simulink model "ME322_Exercise_3_Traction_Motor_Simulink"  (R2024b)
settings: Solver=VariableStepAuto  StartTime=0.0  StopTime=0.025  RelTol=1e-3
undefined symbols (not defined in the file or in its folder): u_trac, x_trac
settings Model: Creator=caidenbonney  LastModifiedBy=Caide

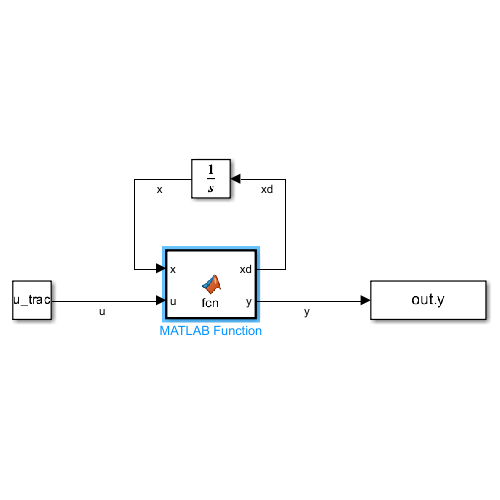
[thumbnail: Simulink's stored preview of the top-level diagram]
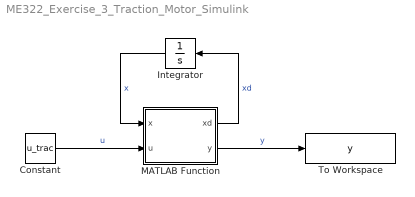
== system ME322_Exercise_3_Traction_Motor_Simulink ==
  Constant : Constant  Value=u_trac  VectorParams1D=off
  Integrator : Integrator  InitialCondition=x_trac
  MATLAB Function : MATLAB Function  TreatAsAtomicUnit=on
  To Workspace : ToWorkspace  VariableName=y  SampleTime=-1
  wires:
  Constant/1 -> MATLAB Function/2(u)  "u"
  MATLAB Function/1(xd) -> Integrator/1  "xd"
  Integrator/1 -> MATLAB Function/1(x)  "x"
  MATLAB Function/2(y) -> To Workspace/1  "y"

== matlab function ME322_Exercise_3_Traction_Motor_Simulink/MATLAB Function ==
  data: x input; xd output size=3; u input; y output size=6; p parameter
function [xd, y]= fcn(x, u, p)

% Separate state variables into individual elements
i_Lm = x(1);     % [A]
omega_Je = x(2); % [rad/sec]
V_me = x(3);    % [m/s]

% Separate input variables into individual elements
v_m = u(1); % [V]

% Required given constants units
p.r_w; % [m]

p.mu_k; % [-]
p.m_e; % [kg]
g = 9.81; % [m/sec^2] (gravity)
p.k; % [-]
p.v_hat; % [m/sec]

p.v_hat; % [m/sec]

p.L_m; % [mH]
L_m = p.L_m *10^-3;  % [mH] -> 10^-3 [H]
p.R_m; % [ohms]
p.K_v; % [V*sec/rad]

p.J_e; % [g/mm^2]
J_e = p.J_e *10^-9;  % [g*mm^2] -> 10^-9 [rad/sec^2)/N*m]^-1
p.K_t; % [N*m/A]
p.b_g; % [N*m/sec]
p.b_m; % [N*m/sec]
p.r_w; % [m]

p.m_e; % [kg]

% Output Equations
V_btr = p.r_w*omega_Je - V_me; % [m/sec]

F_max = p.mu_k*p.m_e*g; % [N]
F_btr = ((2*F_max)/pi)*atan((tan((pi*p.k)/2)/p.v_hat)*V_btr); % [N]

alpha_btr = abs(V_btr) >= p.v_hat; % [-]

% State Equations
id_Lm = (1/(L_m))*(v_m - p.R_m*i_Lm - p.K_v*(p.N_G/p.N_P)*omega_Je); % <-- State eq. f_1
    % the expected units of the derivative of current with respect to
    % time is [A/sec]
        % (1/[H])    *    ([V] - [ohms]*[A] - [V*sec/rad]*[rad/sec])
        % (1/[V/(A/sec)])*([V] -  [V/A]*[A] - [V*sec/rad]*[rad/sec])
        % ([(A/sec)/V]  * ([V] - [V] - [V])
        % ([(A/sec)/V)*[V]
        % [A/sec]

omegad_Je = (1/J_e)*(-p.b_g*omega_Je - (p.N_G/p.N_P)*(p.b_m*(p.N_G/p.N_P)*omega_Je - p.K_t*i_Lm) - p.r_w*F_btr); % <-- State eq. f_2
    % the expected units of the derivative of rotational speed with respect
    % to time is [rad/sec^2]
        % (1/([rad/sec^2)/N*m]^-1))*(-[N*m/sec]*[rad/sec]-([N*m/sec]*[rad/sec]+[N*m/A]*[A]) + [m]*[N])
        % ([rad/sec^2)/N*m])    *   (-[N*m] - ([N*m] + [N*m]) - [N*m])
        % ([rad/sec^2)/N*m])*[N*m]
        % [rad/sec^2]

Vd_me = (1/p.m_e)*F_btr; % <-- State eq. f_3
    % the expected units of the derivative of speed with respect to
    % time is [m/sec^2]
        % (1/[kg])*[N]
        % (1/[kg])*[kg*(m/sec^2)]
        % [m/sec^2]

xd = [id_Lm     % <-- State f_1 [A/sec]
      omegad_Je % <-- State f_2 [rad/sec^2]
      Vd_me];   % <-- State f_3 [m/sec^2]

y = [i_Lm        % <-- Output g_1 [A]
     omega_Je    % <-- Output g_2 [rad/sec]
     V_me        % <-- Output g_3 [m/sec]
     V_btr       % <-- Output g_4 [m/sec]
     F_btr       % <-- Output g_5 [N]
     alpha_btr]; % <-- Output g_6 [-]
